simulink model "Mask"  (R2023b)
settings: Solver=VariableStepAuto  StartTime=0.0  StopTime=28  RelTol=1e-3
libraries: simulink x3, robotmobilelib x1
settings Model: Creator=rubencruzgonzalez  LastModifiedBy=rubencruzgonzalez

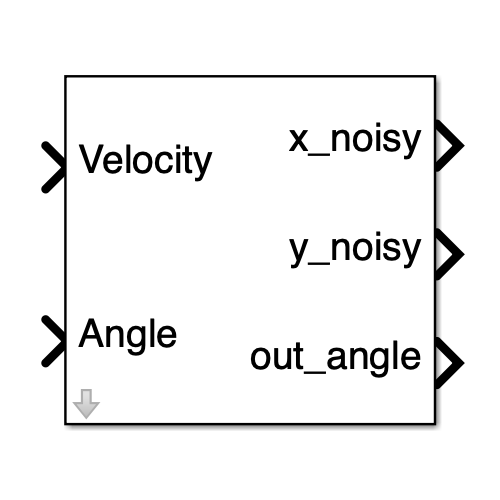
[thumbnail: Simulink's stored preview of the top-level diagram]
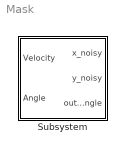
== system Mask ==
  Subsystem : Subsystem

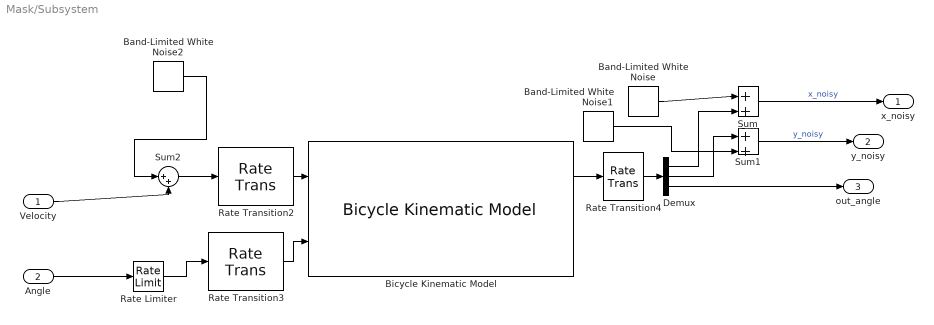
== system Mask/Subsystem ==
  Velocity : Inport
  Angle : Inport  Port=2
  Band-Limited White Noise : simulink/Sources/Band-Limited White Noise  Tag=noise_x  Cov=[0.01]  Ts=1/100  seed=[23341]
  Band-Limited White Noise1 : simulink/Sources/Band-Limited White Noise  Tag=noise_y  Cov=[0.01]  Ts=1/100  seed=[23341]
  Band-Limited White Noise2 : simulink/Sources/Band-Limited White Noise  Tag=noise_x  Cov=[0.001]  Ts=1/100000  seed=[23341]
  Bicycle Kinematic Model : robotmobilelib/Bicycle Kinematic Model  VehicleInputs=Vehicle Speed & Steering Angle  WheelBase=1  VehicleSpeedRange=[0 30]  MaxSteeringAngle=pi/4  InitialState=[0; 0; 0]  SimulateUsing=Code generation
  Demux : Demux  Outputs=3
  Rate Limiter : RateLimiter  RisingSlewLimit=pi/4  FallingSlewLimit=-pi/4  SampleTimeMode=inherited
  Rate Transition2 : RateTransition  OutPortSampleTime=1/1000
  Rate Transition3 : RateTransition  OutPortSampleTime=1/1000
  Rate Transition4 : RateTransition  OutPortSampleTime=1/1000
  Sum : Sum  Inputs=|++
  Sum1 : Sum  Inputs=|++
  Sum2 : Sum  Inputs=|++
  x_noisy : Outport
  y_noisy : Outport  Port=2
  out_angle : Outport  Port=3
  wires:
  Rate Transition2/1 -> Bicycle Kinematic Model/1
  Rate Limiter/1 -> Rate Transition3/1
  Band-Limited White Noise1/1 -> Sum1/2
  Rate Transition3/1 -> Bicycle Kinematic Model/2
  Demux/2 -> Sum1/1
  Band-Limited White Noise/1 -> Sum/1
  Demux/3 -> out_angle/1
  Sum1/1 -> y_noisy/1  "y_noisy"
  Sum2/1 -> Rate Transition2/1
  Band-Limited White Noise2/1 -> Sum2/1
  Sum/1 -> x_noisy/1  "x_noisy"
  Rate Transition4/1 -> Demux/1
  Angle/1 -> Rate Limiter/1
  Demux/1 -> Sum/2
  Bicycle Kinematic Model/1 -> Rate Transition4/1
  Velocity/1 -> Sum2/2
